simulink model "gain_test_ElementWise_complex"  (Simulink 8.4)
settings: Solver=ode3  StartTime=0.0  StopTime=10.0  FixedStep=0.1  RelTol=1e-3
settings Model: Creator=arnaud  LastModifiedBy=arnaud
settings DataIOCC: SaveFormat=Structure
settings DebuggingCC: UnnecessaryDatatypeConvMsg=warning  VectorMatrixConversionMsg=warning

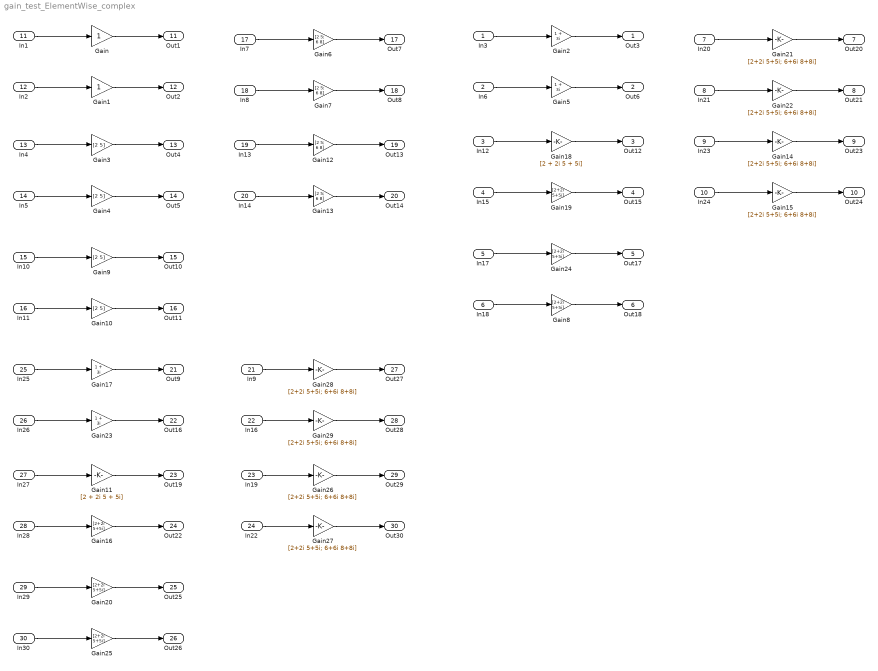
== system gain_test_ElementWise_complex ==
  In3 : Inport  OutDataTypeStr=double
  In6 : Inport  Port=2  OutDataTypeStr=int8
  In12 : Inport  Port=3  OutDataTypeStr=double  PortDimensions=1
  In15 : Inport  Port=4  OutDataTypeStr=int8  PortDimensions=1
  In17 : Inport  Port=5  OutDataTypeStr=double  PortDimensions=2
  In18 : Inport  Port=6  OutDataTypeStr=int8  PortDimensions=2
  In20 : Inport  Port=7  OutDataTypeStr=double  PortDimensions=1
  In21 : Inport  Port=8  OutDataTypeStr=int8  PortDimensions=1
  In23 : Inport  Port=9  OutDataTypeStr=double  PortDimensions=[2 2]
  In24 : Inport  Port=10  OutDataTypeStr=int8  PortDimensions=[2 2]
  In1 : Inport  Port=11  OutDataTypeStr=double
      settings: SignalType=complex
  In2 : Inport  Port=12  OutDataTypeStr=int8
      settings: SignalType=complex
  In4 : Inport  Port=13  OutDataTypeStr=double  PortDimensions=1
      settings: SignalType=complex
  In5 : Inport  Port=14  OutDataTypeStr=int8  PortDimensions=1
      settings: SignalType=complex
  In10 : Inport  Port=15  OutDataTypeStr=double  PortDimensions=2
      settings: SignalType=complex
  In11 : Inport  Port=16  OutDataTypeStr=int8  PortDimensions=2
      settings: SignalType=complex
  In7 : Inport  Port=17  OutDataTypeStr=double  PortDimensions=1
      settings: SignalType=complex
  In8 : Inport  Port=18  OutDataTypeStr=int8  PortDimensions=1
      settings: SignalType=complex
  In13 : Inport  Port=19  OutDataTypeStr=double  PortDimensions=[2 2]
      settings: SignalType=complex
  In14 : Inport  Port=20  OutDataTypeStr=int8  PortDimensions=[2 2]
      settings: SignalType=complex
  In9 : Inport  Port=21  OutDataTypeStr=double  PortDimensions=1
      settings: SignalType=complex
  In16 : Inport  Port=22  OutDataTypeStr=int8  PortDimensions=1
      settings: SignalType=complex
  In19 : Inport  Port=23  OutDataTypeStr=double  PortDimensions=[2 2]
      settings: SignalType=complex
  In22 : Inport  Port=24  OutDataTypeStr=int8  PortDimensions=[2 2]
      settings: SignalType=complex
  In25 : Inport  Port=25  OutDataTypeStr=double
      settings: SignalType=complex
  In26 : Inport  Port=26  OutDataTypeStr=int8
      settings: SignalType=complex
  In27 : Inport  Port=27  OutDataTypeStr=double  PortDimensions=1
      settings: SignalType=complex
  In28 : Inport  Port=28  OutDataTypeStr=int8  PortDimensions=1
      settings: SignalType=complex
  In29 : Inport  Port=29  OutDataTypeStr=double  PortDimensions=2
      settings: SignalType=complex
  In30 : Inport  Port=30  OutDataTypeStr=int8  PortDimensions=2
      settings: SignalType=complex
  Gain : Gain
  Gain1 : Gain
  Gain{3..4,9..10} (4 alike) : Gain  Gain=[2 5]
  Gain11 : Gain  Gain=[2 + 2i 5 + 5i]
  Gain{6..7,12..13} (4 alike) : Gain  Gain=[2 5; 6 8]
  Gain{14..15,21..22,26..29} (8 alike) : Gain  Gain=[2+2i 5+5i; 6+6i 8+8i]
  Gain{8,16,19..20,24..25} (6 alike) : Gain  Gain=[2+2i 5+5i]
  Gain{2,5,17,23} (4 alike) : Gain  Gain=1 + 3i
  Gain18 : Gain  Gain=[2 + 2i 5 + 5i]
  Out3 : Outport
  Out6 : Outport  Port=2
  Out12 : Outport  Port=3
  Out15 : Outport  Port=4
  Out17 : Outport  Port=5
  Out18 : Outport  Port=6
  Out20 : Outport  Port=7
  Out21 : Outport  Port=8
  Out23 : Outport  Port=9
  Out24 : Outport  Port=10
  Out1 : Outport  Port=11
  Out2 : Outport  Port=12
  Out4 : Outport  Port=13
  Out5 : Outport  Port=14
  Out10 : Outport  Port=15
  Out11 : Outport  Port=16
  Out7 : Outport  Port=17
  Out8 : Outport  Port=18
  Out13 : Outport  Port=19
  Out14 : Outport  Port=20
  Out9 : Outport  Port=21
  Out16 : Outport  Port=22
  Out19 : Outport  Port=23
  Out22 : Outport  Port=24
  Out25 : Outport  Port=25
  Out26 : Outport  Port=26
  Out27 : Outport  Port=27
  Out28 : Outport  Port=28
  Out29 : Outport  Port=29
  Out30 : Outport  Port=30
  wires:
  In3/1 -> Gain2/1
  Gain2/1 -> Out3/1
  In6/1 -> Gain5/1
  Gain5/1 -> Out6/1
  In12/1 -> Gain18/1
  Gain18/1 -> Out12/1
  In15/1 -> Gain19/1
  Gain19/1 -> Out15/1
  In17/1 -> Gain24/1
  Gain24/1 -> Out17/1
  In18/1 -> Gain8/1
  Gain8/1 -> Out18/1
  In20/1 -> Gain21/1
  Gain21/1 -> Out20/1
  In21/1 -> Gain22/1
  Gain22/1 -> Out21/1
  In23/1 -> Gain14/1
  Gain14/1 -> Out23/1
  In24/1 -> Gain15/1
  Gain15/1 -> Out24/1
  In1/1 -> Gain/1
  Gain/1 -> Out1/1
  In2/1 -> Gain1/1
  Gain1/1 -> Out2/1
  In4/1 -> Gain3/1
  Gain3/1 -> Out4/1
  In5/1 -> Gain4/1
  Gain4/1 -> Out5/1
  In10/1 -> Gain9/1
  Gain9/1 -> Out10/1
  In11/1 -> Gain10/1
  Gain10/1 -> Out11/1
  In7/1 -> Gain6/1
  Gain6/1 -> Out7/1
  In8/1 -> Gain7/1
  Gain7/1 -> Out8/1
  In13/1 -> Gain12/1
  Gain12/1 -> Out13/1
  In14/1 -> Gain13/1
  Gain13/1 -> Out14/1
  In25/1 -> Gain17/1
  Gain17/1 -> Out9/1
  In26/1 -> Gain23/1
  Gain23/1 -> Out16/1
  In27/1 -> Gain11/1
  Gain11/1 -> Out19/1
  In28/1 -> Gain16/1
  Gain16/1 -> Out22/1
  In29/1 -> Gain20/1
  Gain20/1 -> Out25/1
  In30/1 -> Gain25/1
  Gain25/1 -> Out26/1
  In9/1 -> Gain28/1
  Gain28/1 -> Out27/1
  In16/1 -> Gain29/1
  Gain29/1 -> Out28/1
  In19/1 -> Gain26/1
  Gain26/1 -> Out29/1
  In22/1 -> Gain27/1
  Gain27/1 -> Out30/1
